simulink model "test_hueseyin"  (R2017a)
settings: Solver=VariableStepAuto  StartTime=0.0  StopTime=10.0  RelTol=1e-3
settings Model: Creator=DeltaRacing  LastModifiedBy=DeltaRacing

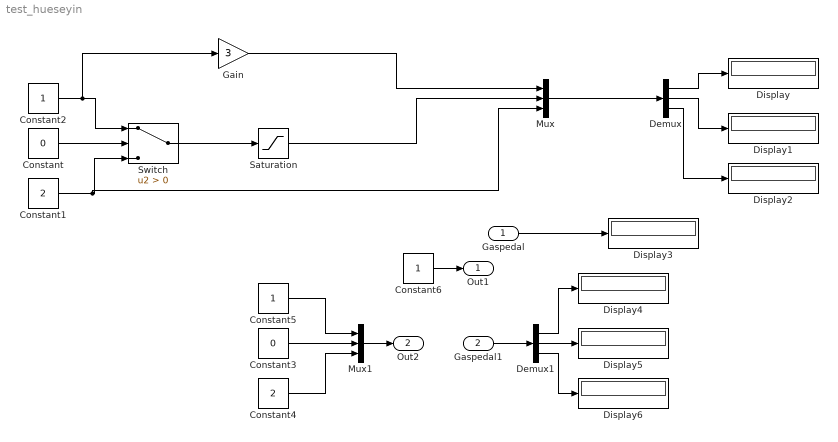
== system test_hueseyin ==
  Gaspedal : Inport  Interpolate=off
  Gaspedal1 : Inport  Port=2  Interpolate=off
  Constant : Constant  Value=0
  Constant1 : Constant  Value=2
  Constant2 : Constant
  Constant3 : Constant  Value=0
  Constant4 : Constant  Value=2
  Constant5 : Constant
  Constant6 : Constant
  Demux : Demux  Outputs=3
  Demux1 : Demux  Outputs=3
  Display{,1..6} (7 alike) : Display
  Gain : Gain  Gain=3
  Mux : Mux  Inputs=3
  Mux1 : Mux  Inputs=3
  Saturation : Saturate  UpperLimit=1.5
  Switch : Switch  Criteria=u2 > Threshold
  "Out1 " : Outport
  Out2 : Outport  Port=2
  wires:
  Constant2/1 -> Gain/1, Switch/1
  Demux/1 -> Display/1
  Constant/1 -> Switch/2
  Demux/2 -> Display1/1
  Saturation/1 -> Mux/2
  Constant1/1 -> Mux/3, Switch/3
  Gain/1 -> Mux/1
  Switch/1 -> Saturation/1
  Mux/1 -> Demux/1
  Constant4/1 -> Mux1/3
  Constant3/1 -> Mux1/2
  Mux1/1 -> Out2/1
  Demux/3 -> Display2/1
  Constant5/1 -> Mux1/1
  Constant6/1 -> "Out1 "/1
  Gaspedal/1 -> Display3/1
  Gaspedal1/1 -> Demux1/1
  Demux1/2 -> Display5/1
  Demux1/1 -> Display4/1
  Demux1/3 -> Display6/1
